simulink model "OcularMotorLabModel"  (R2023a)
settings: Solver=FixedStepAuto  StartTime=tStart  StopTime=tFinal  FixedStep=0.001  RelTol=1e-3
undefined symbols (not defined in the file or in its folder): Asp, Asp1, Asp2, e0sp, gaussian, Gpc, GPos, Gsl, HeadToEye, IPD, psi, Psp1, RotFbk, SacThDeg, SatSp, sigbuilder_block, SomFbk, T1, T2, Tccanal, Tcn, Tcr, Tcsp, TCvs, tdm, tdsp1, tdsp2, tdsp3, tdv, Tsl, Tz, w
libraries: matrix_library x16, vrlib x9, simulink_extras x8, simulink x1
(part 3 of 3)

== system OcularMotorLabModel/Visual World Intrinsic velocity/Subsystem ==
  In1 : Inport
  Demux : Demux  Tag=STV Demux  Outputs=3
      settings: DisplayOption=none
  N-O (roll) : Outport  Tag=STV Outport
  I-A (pitch) : Outport  Tag=STV Outport  Port=2
  R-C (yaw) : Outport  Tag=STV Outport  Port=3
  wires:
  Demux/1 -> N-O (roll)/1
  Demux/2 -> I-A (pitch)/1
  Demux/3 -> R-C (yaw)/1
  In1/1 -> Demux/1

== system OcularMotorLabModel/Visual linear world extrinsic velocity/Subsystem ==
  In1 : Inport
  Demux : Demux  Tag=STV Demux  Outputs=3
      settings: DisplayOption=none
  vx : Outport  Tag=STV Outport
  vy : Outport  Tag=STV Outport  Port=2
  vz : Outport  Tag=STV Outport  Port=3
  wires:
  Demux/1 -> vx/1
  Demux/2 -> vy/1
  Demux/3 -> vz/1
  In1/1 -> Demux/1

== system OcularMotorLabModel/Visual linear world intrinsic velocity/Subsystem ==
  In1 : Inport
  Demux : Demux  Tag=STV Demux  Outputs=3
      settings: DisplayOption=none
  vX : Outport  Tag=STV Outport
  vY : Outport  Tag=STV Outport  Port=2
  vZ : Outport  Tag=STV Outport  Port=3
  wires:
  Demux/1 -> vX/1
  Demux/2 -> vY/1
  Demux/3 -> vZ/1
  In1/1 -> Demux/1

== system OcularMotorLabModel/Smooth pursuit/Internal model/Eye plant ==
  In1 : Inport
  Demux : Demux  Outputs=3
  Mux : Mux  Inputs=3
  Plant1 : TransferFcn  Numerator=[Tz 1]  Denominator=[T1*T2 (T1+T2) 1]
  Plant2 : TransferFcn  Numerator=[w^2]  Denominator=[1 + 2*psi*w w^2]
  Plant3 : TransferFcn  Numerator=[Tz 1]  Denominator=[T1*T2 (T1+T2) 1]
  Plant4 : TransferFcn  Numerator=[w^2]  Denominator=[1 + 2*psi*w w^2]
  Plant5 : TransferFcn  Numerator=[Tz 1]  Denominator=[T1*T2 (T1+T2) 1]
  Plant6 : TransferFcn  Numerator=[w^2]  Denominator=[1 + 2*psi*w w^2]
  Eye position : Outport
  wires:
  In1/1 -> Demux/1
  Mux/1 -> Eye position/1  "Eye position"
  Plant4/1 -> Mux/1
  Plant2/1 -> Mux/2
  Plant6/1 -> Mux/3
  Demux/1 -> Plant3/1
  Demux/2 -> Plant1/1
  Demux/3 -> Plant5/1
  Plant3/1 -> Plant4/1
  Plant1/1 -> Plant2/1
  Plant5/1 -> Plant6/1
